simulink model "ODE_Hand_Model_v04"  (Simulink 7.5)
settings: Solver=ode1  StartTime=0.0  StopTime=inf  FixedStep=0.0315/(3*12)  RelTol=1e-3
settings Model: Creator=nihil  LastModifiedBy=konstantinos

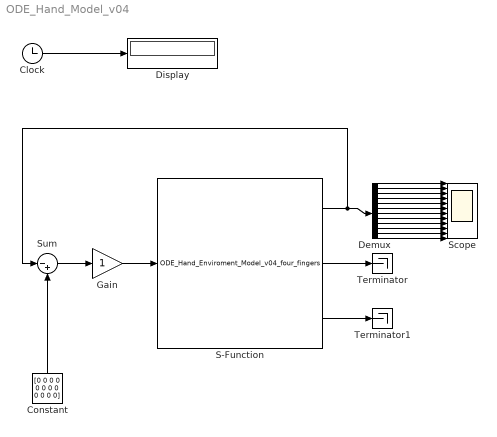
== system ODE_Hand_Model_v04 ==
  Clock : Clock
      settings: Decimation=10
  Constant : Constant  Value=[0 0 0 0 0 0 0 0 0 0 0 0]  OutDataType=fixdt(1, 16)  OutScaling=2^0
  Demux : Demux  Outputs=12
  Display : Display
  Gain : Gain  ParameterDataType=fixdt(1, 16)  ParameterScaling=2^0  OutDataType=fixdt(1, 16)  OutScaling=2^0
  S-Function : S-Function  FunctionName=ODE_Hand_Enviroment_Model_v04_four_fingers  EnableBusSupport=off
  Scope : Scope  NumInputPorts=12
      settings: TimeRange=3.418747299743785e-005  YMin=0.2719907407407408~-1~-1~0~0~-4e-010~0~-2e-015~-4e-010~-1~-1~-1  YMax=0.3020833333333333~1~1~2~2e-015~0~2~2e-015~0~1~1~1
  Sum : Sum  Inputs=|-+  OutDataType=fixdt(1, 16)  OutScaling=2^0
  Terminator : Terminator
  Terminator1 : Terminator
  wires:
  Clock/1 -> Display/1
  Constant/1 -> Sum/2
  S-Function/1 -> Demux/1, Sum/1
  Sum/1 -> Gain/1
  Gain/1 -> S-Function/1
  Demux/1 -> Scope/1
  Demux/2 -> Scope/2
  Demux/3 -> Scope/3
  Demux/4 -> Scope/4
  Demux/5 -> Scope/5
  Demux/6 -> Scope/6
  Demux/7 -> Scope/7
  Demux/8 -> Scope/8
  Demux/9 -> Scope/9
  Demux/10 -> Scope/10
  Demux/11 -> Scope/11
  Demux/12 -> Scope/12
  S-Function/2 -> Terminator/1
  S-Function/3 -> Terminator1/1
